simulink model "dsp_proj_v2_2024"  (R2024b)
settings: Solver=FixedStepDiscrete  StartTime=0.0  StopTime=1e-4  FixedStep=1/60e6  RelTol=1e-3
libraries: hdlsllib x12, simulink x4, dspfdesign x3
settings Model: Creator=UTSAB KARAN  LastModifiedBy=souma
settings ConfigComp: CovBoundaryAbsTol=1.0e-5

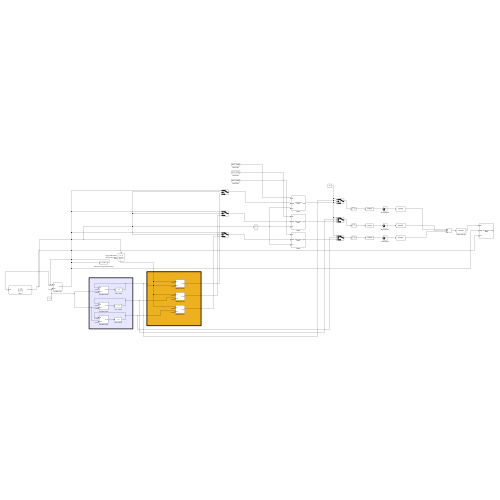
[thumbnail: Simulink's stored preview of the top-level diagram]
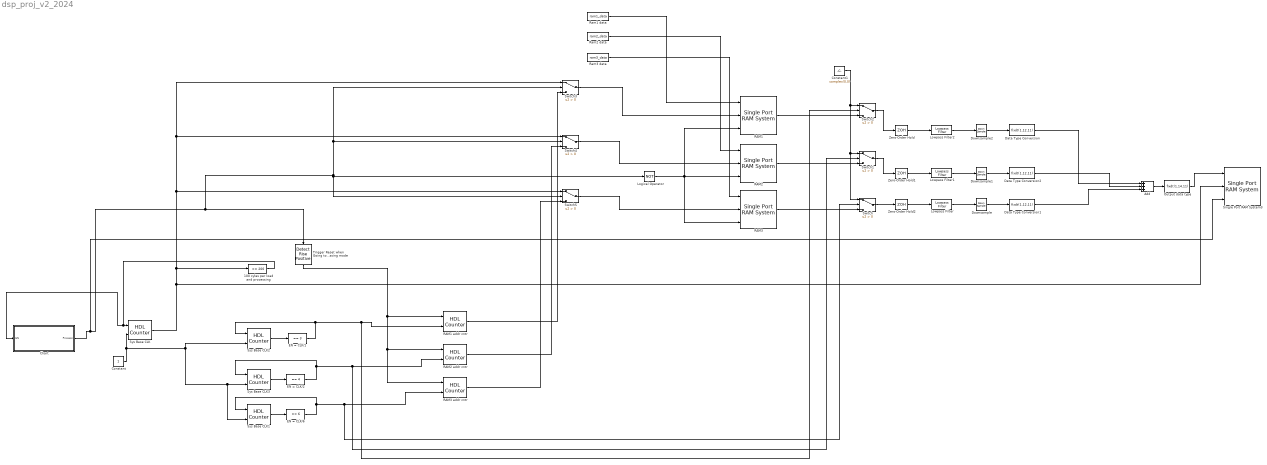
== system dsp_proj_v2_2024 ==
  100 cyles per load and processing : simulink/Logic and Bit Operations/Compare To Constant  relop===  const=200  OutDataTypeStr=boolean
  Add : Sum  Inputs=+++
  Chart : Stateflow chart  TreatAsAtomicUnit=on
  Constant : Constant  OutDataTypeStr=boolean
  Constant1 : Constant  Value=complex(0,0)  VectorParams1D=off  SampleTime=-1  LockScale=on
  Data Type Conversion : DataTypeConversion  OutDataTypeStr=fixdt(1,12,11)  SaturateOnIntegerOverflow=off  RndMeth=Floor
  Data Type Conversion1 : DataTypeConversion  OutDataTypeStr=fixdt(1,12,11)  SaturateOnIntegerOverflow=off  RndMeth=Floor
  Data Type Conversion2 : DataTypeConversion  OutDataTypeStr=fixdt(1,12,11)  SaturateOnIntegerOverflow=off  RndMeth=Floor
  Downsample : DownSample  N=5  RateOptions=Allow multirate processing
  Downsample1 : DownSample  N=5  RateOptions=Allow multirate processing
  Downsample2 : DownSample  N=5  RateOptions=Allow multirate processing
  EN = CLK/1 : simulink/Logic and Bit Operations/Compare To Constant  relop===  const=3  OutDataTypeStr=boolean
  EN = CLK/2 : simulink/Logic and Bit Operations/Compare To Constant  relop===  const=4  OutDataTypeStr=boolean
  EN = CLK/6 : simulink/Logic and Bit Operations/Compare To Constant  relop===  const=6  OutDataTypeStr=boolean
  Logical Operator : Logic  Operator=NOT  AllPortsSameDT=off  OutDataTypeStr=boolean
  Lowpass Filter : dspfdesign/Lowpass Filter  FilterType=FIR  DesignForMinimumOrder=on  FilterOrder=50  PassbandFrequency=0.4  StopbandFrequency=0.5  PassbandRipple=0.1  StopbandAttenuation=80  SampleRateMode=Use normalized frequency (0 to 1)  SampleRate=60e6  SimulateUsing=Interpreted execution  roundingMode=Floor  coeffsDataTypeStr=fixdt(1,16,15)
  Lowpass Filter1 : dspfdesign/Lowpass Filter  FilterType=FIR  DesignForMinimumOrder=on  FilterOrder=50  PassbandFrequency=0.4  StopbandFrequency=0.5  PassbandRipple=0.1  StopbandAttenuation=80  SampleRateMode=Use normalized frequency (0 to 1)  SampleRate=60e6  SimulateUsing=Interpreted execution  roundingMode=Floor  coeffsDataTypeStr=fixdt(1,16,15)
  Lowpass Filter2 : dspfdesign/Lowpass Filter  FilterType=FIR  DesignForMinimumOrder=on  FilterOrder=50  PassbandFrequency=0.4  StopbandFrequency=0.5  PassbandRipple=0.1  StopbandAttenuation=80  SampleRateMode=Use normalized frequency (0 to 1)  SampleRate=60e6  SimulateUsing=Interpreted execution  roundingMode=Floor  coeffsDataTypeStr=fixdt(1,16,15)
  Output data type : DataTypeConversion  OutDataTypeStr=fixdt(1,14,11)  SaturateOnIntegerOverflow=off  RndMeth=Floor  LockScale=on
  RAM1 : hdlsllib/HDL RAMs/Single Port RAM System  RAMType=Single port  AsyncRead=off  WriteOutputValue=New data  RAMInitialValue=0  allowBusInputs=off  WritesHaveOutput=on  NumReads=0  NumWrites=1  SimulateUsing=Code generation  ModelRAMDelay=on  VectorAccess=Parallel
  RAM1 addr cntr : hdlsllib/Sources/HDL Counter  CountType=Count limited  CountInit=0  CountStep=1  CountMax=1000  CountFromType=Initial value  CountFrom=0  CountResetPort=on  CountLoadPort=off  CountEnbPort=on  CountDirPort=off  CountHitOutputPort=off  CountDataType=Unsigned  CountWordLen=12  CountFracLen=0  CountSampTime=1
  RAM2 : hdlsllib/HDL RAMs/Single Port RAM System  RAMType=Single port  AsyncRead=off  WriteOutputValue=New data  RAMInitialValue=0  allowBusInputs=off  WritesHaveOutput=on  NumReads=0  NumWrites=1  SimulateUsing=Code generation  ModelRAMDelay=on  VectorAccess=Parallel
  RAM2 addr cntr : hdlsllib/Sources/HDL Counter  CountType=Count limited  CountInit=0  CountStep=1  CountMax=1000  CountFromType=Initial value  CountFrom=0  CountResetPort=on  CountLoadPort=off  CountEnbPort=on  CountDirPort=off  CountHitOutputPort=off  CountDataType=Unsigned  CountWordLen=12  CountFracLen=0  CountSampTime=1
  RAM3 : hdlsllib/HDL RAMs/Single Port RAM System  RAMType=Single port  AsyncRead=off  WriteOutputValue=New data  RAMInitialValue=0  allowBusInputs=off  WritesHaveOutput=on  NumReads=0  NumWrites=1  SimulateUsing=Code generation  ModelRAMDelay=on  VectorAccess=Parallel
  RAM3 addr cntr : hdlsllib/Sources/HDL Counter  CountType=Count limited  CountInit=0  CountStep=1  CountMax=1000  CountFromType=Initial value  CountFrom=0  CountResetPort=on  CountLoadPort=off  CountEnbPort=on  CountDirPort=off  CountHitOutputPort=off  CountDataType=Unsigned  CountWordLen=12  CountFracLen=0  CountSampTime=1
  Ram1 data : FromWorkspace  VariableName=ram1_data  Interpolate=off  OutputAfterFinalValue=Holding final value
  Ram2 data : FromWorkspace  VariableName=ram2_data  Interpolate=off  OutputAfterFinalValue=Holding final value
  Ram3 data : FromWorkspace  VariableName=ram3_data  Interpolate=off  OutputAfterFinalValue=Holding final value
  Single Port RAM System3 : hdlsllib/HDL RAMs/Single Port RAM System  RAMType=Single port  AsyncRead=off  WriteOutputValue=New data  RAMInitialValue=0  allowBusInputs=off  WritesHaveOutput=on  NumReads=0  NumWrites=1  SimulateUsing=Code generation  ModelRAMDelay=on  VectorAccess=Parallel
  Switch{,1..5} (6 alike) : Switch  Criteria=u2 > Threshold  SaturateOnIntegerOverflow=off  InputSameDT=off
  Sys Base CLK{,1..3} (4 alike) : hdlsllib/Sources/HDL Counter  CountType=Count limited  CountInit=0  CountStep=1  CountMax=1000  CountFromType=Initial value  CountFrom=0  CountResetPort=on  CountLoadPort=off  CountEnbPort=on  CountDirPort=off  CountHitOutputPort=off  CountDataType=Unsigned  CountWordLen=12  CountFracLen=0  CountSampTime=1
  Trigger Reset when Going to processing mode : hdlsllib/Logic and Bit Operations/Detect Rise Positive  vinit=0  OutDataTypeStr=boolean
  Zero-Order Hold : ZeroOrderHold  SampleTime=1/10e6
  Zero-Order Hold1 : ZeroOrderHold  SampleTime=1/15e6
  Zero-Order Hold2 : ZeroOrderHold  SampleTime=1/20e6
  wires:
  Sys Base CLK/1 -> Single Port RAM System3/2, 100 cyles per load and processing/1, Switch5/1, Switch3/1, Switch4/1
  Constant/1 -> Sys Base CLK3/2, Sys Base CLK1/2, Sys Base CLK2/2, Sys Base CLK/2
  100 cyles per load and processing/1 -> Chart/1(EN), Sys Base CLK/1
  EN = CLK/6/1 -> Sys Base CLK1/1, RAM3 addr cntr/2, Switch/2
  RAM1 addr cntr/1 -> Switch3/3
  RAM2 addr cntr/1 -> Switch4/3
  RAM3 addr cntr/1 -> Switch5/3
  Switch1/1 -> Zero-Order Hold1/1
  Add/1 -> Output data type/1
  Output data type/1 -> Single Port RAM System3/1
  Chart/1(Process) -> Single Port RAM System3/3, Switch5/2, Logical Operator/1, Switch3/2, Switch4/2, Trigger Reset when Going to processing mode/1
  Ram1 data/1 -> RAM1/1
  Ram2 data/1 -> RAM2/1
  Ram3 data/1 -> RAM3/1
  Trigger Reset when Going to processing mode/1 -> RAM1 addr cntr/1, RAM3 addr cntr/1, RAM2 addr cntr/1
  RAM1/1 -> Switch2/3
  Constant1/1 -> Switch/1, Switch1/1, Switch2/1
  Switch3/1 -> RAM1/2
  Switch4/1 -> RAM2/2
  Sys Base CLK1/1 -> EN = CLK/6/1
  Sys Base CLK2/1 -> EN = CLK/1/1
  EN = CLK/2/1 -> Sys Base CLK3/1, RAM2 addr cntr/2, Switch1/2
  Sys Base CLK3/1 -> EN = CLK/2/1
  Switch5/1 -> RAM3/2
  Logical Operator/1 -> RAM1/3, RAM2/3, RAM3/3
  EN = CLK/1/1 -> RAM1 addr cntr/2, Switch2/2, Sys Base CLK2/1
  RAM2/1 -> Switch1/3
  RAM3/1 -> Switch/3
  Switch/1 -> Zero-Order Hold2/1
  Switch2/1 -> Zero-Order Hold/1
  Lowpass Filter2/1 -> Downsample2/1
  Lowpass Filter1/1 -> Downsample1/1
  Lowpass Filter/1 -> Downsample/1
  Zero-Order Hold/1 -> Lowpass Filter2/1
  Zero-Order Hold1/1 -> Lowpass Filter1/1
  Zero-Order Hold2/1 -> Lowpass Filter/1
  Downsample2/1 -> Data Type Conversion/1
  Downsample1/1 -> Data Type Conversion2/1
  Downsample/1 -> Data Type Conversion1/1
  Data Type Conversion1/1 -> Add/3
  Data Type Conversion2/1 -> Add/2
  Data Type Conversion/1 -> Add/1

== stateflow chart dsp_proj_v2_2024/Chart ==
  settings: stateMachineType=MOORE_MACHINE  executeAtInitialization=1
  state Processing
    Process = true
  state Data_Loading
    Process = false
  Data_Loading -> Processing : [ EN==1]
  (default) -> Data_Loading
  data: Process output; EN input
